simulink model "turboShaft_Harness1"  (R2024a)
settings: Solver=VariableStepAuto  StartTime=0.0  StopTime=1000  RelTol=1e-3
model workspace: external: MATLAB File C:\Users\imyrsini\OneDrive - MathWorks\Documents\Projects\AEprojects\LSTM Model Reduction\turboShaftEngine\initialization.m (data not in the file)
undefined symbols (not defined in the file): burner, height
libraries: fl_lib x1, simulink x1, nesl_utility x1
settings Model: Creator=imyrsini  LastModifiedBy=imyrsini
settings RTWCC: GPUComputeCapability=3.5
settings SimscapeCC: SimscapeLogType=all  SimscapeLogSimulationStatistics=on  SimscapeLogToSDI=on

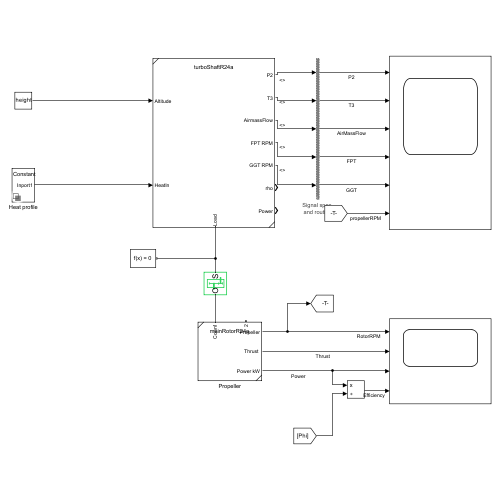
[thumbnail: Simulink's stored preview of the top-level diagram]
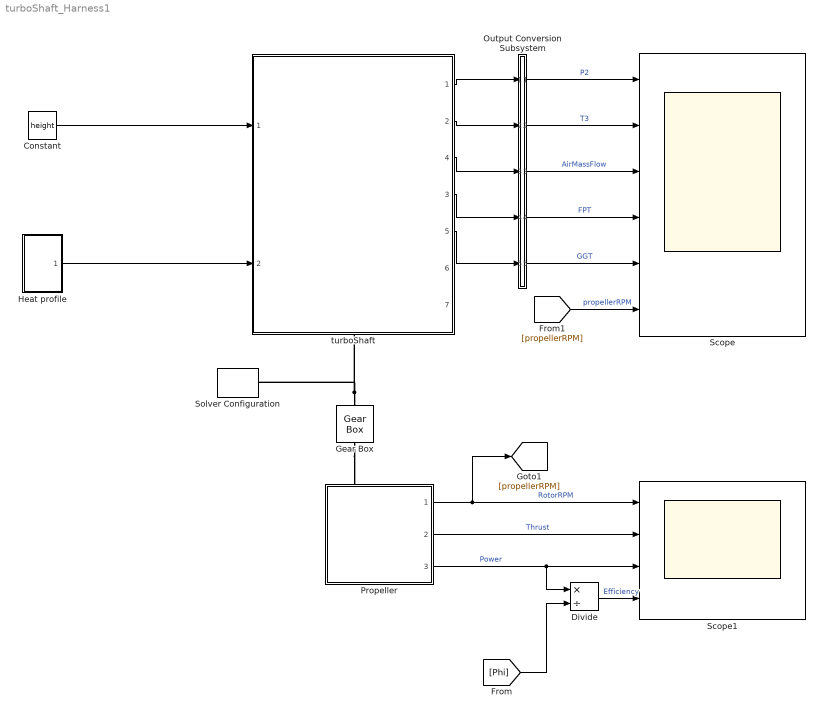
== system turboShaft_Harness1 ==
  Constant : Constant  Value=height
  Divide : Product  Inputs=*/
  Gear Box : fl_lib/Mechanical/Mechanisms/Gear Box  ratio=shaftFTP.GearRatio  t_in_specify=off  t_in_priority=None  t_in=0 N*m  t_in_nominal_specify=off  t_in_nominal_value=1  t_in_nominal_unit=N*m  t_out_specify=off  t_out_priority=None  t_out=0 N*m  t_out_nominal_specify=off  t_out_nominal_value=1  t_out_nominal_unit=N*m
  Heat profile : Subsystem  Variant=on  VariantControlMode=label  VariantControl=Choice  LabelModeActiveChoice=Choice
  Output Conversion Subsystem : Subsystem  Tag=__SLT_OCS__  Description=|
      | Signal spec.
      | and routing
      settings: AttributesFormatString=%<Description>
  Propeller : Subsystem  ReferencedSubsystem=mainRotorR24a
      settings: PortSchema="{\"entries\":[{\"content\":{\"sides\":[{\"content\":{},\"type\":\"ConnectorPlacement.EquallySpacedRectSide\",\"uuid\":\"252db255-f093-4807-9ecd-c68cc83ab3ed\"},{\"content\":{\"connectorIds\":[\"Out1\",\"Out2\",\"Out3\"],\"side\":\"RIGHT\"},\"type\":\"ConnectorPlacement.EquallySpacedRectSide\",\"uuid\":\"da666ad2-6787-4735-89e8-4b014bcd5380\"},{\"content\":{\"connectorIds\":[\"LConn1\",\"LConn2\"],\"side\":\"TOP\"},\"type\":\"ConnectorPlacement.EquallySpacedRectSide\",\"uuid\":\"73693994-4640-4975-b3ef-a4c51496569c\"}]},\"type\":\"ConnectorPlacement.EquallySpacedConnector\",\"uuid\":\"074df9fe-faaf-4ddc-9794-64f4ac4e057a\"}],\"packageUris\":[\"http://schema.mathworks.com/mf0/Connector/R2020b\"],\"version\":\"1.0\"}"
  Scope : Scope  NumInputPorts=6
  Scope1 : Scope  NumInputPorts=4
  Solver Configuration : nesl_utility/Solver Configuration  PhysicalDomain=network_engine_domain  SubClassName=solver  LeftPortType=input  RightPortType=generic  Tones=[]  Harmonics=[]  SimulateNoise=off  Profile=off  UseLocalSampling=off  EnableSwitchedLinearOptims=on  FrequencyDomain=off  UseCCode=off  RelTol=0.001  AbsTol=0.001  MinStep=1e-09  ToWorkspace=off  RevertToSquareIcSolve=off  NumHomotopyIterations=100  PhasorMode=off  PhasorModeNumHarmonics=1  ConsistencySolver=NEWTON_XTOL_AFTER_FTOL  IndexReductionMethod=DerivativeReplacement  DoDC=on  ResidualTolerance=1e-09  ConsistencyTolSource=GLOBAL  ConsistencyAbsTol=0.001  ConsistencyRelTol=0.001  ConsistencyTolFactor=0.001  UseLocalSolver=off  LocalSolverChoice=NE_BACKWARD_EULER_ADVANCER  ResolveIndetEquations=on  FunctionEvalNumThread=1  LocalSolverSampleTime=0.001  DoFixedCost=off  MaxNonlinIter=3  MaxModeIter=2  ComputeImpulses=off  ImpulseIterations=2  LinearAlgebra=auto  LinearAlgebraNumThread=0  EquationFormulation=NE_TIME_EF  DelaysMemoryBudget=1024  AutomaticFiltering=on  FilteringTimeConstant=0.001  PartitionStorageMethod=AS_NEEDED  PartitionMemoryBudget=1024  PartitionMethod=ROBUST  MultibodyUseLocalSolver=off  MultibodyLocalSolverChoice=ODE1  MultibodyLocalSolverSampleTime=0.001
  turboShaft : Subsystem  ReferencedSubsystem=turboShaftR24a
      settings: PortSchema="{\"entries\":[{\"content\":{\"sides\":[{\"content\":{\"connectorIds\":[\"In1\",\"In2\"]},\"type\":\"ConnectorPlacement.EquallySpacedRectSide\",\"uuid\":\"7ef2fcb2-1b0d-44c2-984d-f1d7df0d7e80\"},{\"content\":{\"connectorIds\":[\"Out1\",\"Out2\",\"Out4\",\"Out3\",\"Out5\",\"Out6\",\"Out7\"],\"side\":\"RIGHT\"},\"type\":\"ConnectorPlacement.EquallySpacedRectSide\",\"uuid\":\"b2d8a67b-1c6d-4b5e-865c-86345858511b\"},{\"content\":{\"side\":\"TOP\"},\"type\":\"ConnectorPlacement.EquallySpacedRectSide\",\"uuid\":\"4c7a9b07-6c1b-4859-8cda-a5c2cd89c129\"},{\"content\":{\"connectorIds\":[\"RConn1\"],\"side\":\"BOTTOM\"},\"type\":\"ConnectorPlacement.EquallySpacedRectSide\",\"uuid\":\"794a4e7c-d3e7-4ff8-9cf4-b7022afdc3bd\"}]},\"type\":\"ConnectorPlacement.EquallySpacedConnector\",\"uuid\":\"5f81fd46-9bac-4f96-9ad1-c3a7cd36c01a\"}],\"packageUris\":[\"http://schema.mathworks.com/mf0/Connector/R2020b\"],\"version\":\"1.0\"}"
  wires:
  Output Conversion Subsystem/1(Outport_1) -> Scope/1  "P2"
  Output Conversion Subsystem/2(Outport_2) -> Scope/2  "T3"
  Output Conversion Subsystem/3(Outport_3) -> Scope/3  "AirMassFlow"
  Output Conversion Subsystem/4(Outport_4) -> Scope/4  "FPT"
  Output Conversion Subsystem/5(Outport_5) -> Scope/5  "GGT"
  turboShaft/1 -> Output Conversion Subsystem/1(Inport_1)
  turboShaft/2 -> Output Conversion Subsystem/2(Inport_2)
  turboShaft/4 -> Output Conversion Subsystem/3(Inport_3)
  Propeller/1 -> [propellerRPM], Scope1/1  "RotorRPM"
  Propeller/2 -> Scope1/2  "Thrust"
  Propeller/3 -> Divide/1, Scope1/3  "Power"
  [Phi] -> Divide/2
  Divide/1 -> Scope1/4  "Efficiency"
  turboShaft/3 -> Output Conversion Subsystem/4(Inport_4)
  turboShaft/5 -> Output Conversion Subsystem/5(Inport_5)
  [propellerRPM] -> Scope/6  "propellerRPM"
  Constant/1 -> turboShaft/1
  Heat profile/1(Inport1) -> turboShaft/2
  connections:
  Gear Box/LConn1 -- Solver Configuration/RConn1 -- turboShaft/RConn1
  Gear Box/RConn1 -- Propeller/LConn1

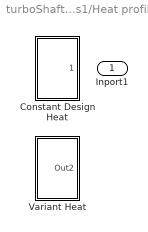
== system turboShaft_Harness1/Heat profile ==
  Constant Design Heat : Subsystem  VariantControl=Choice
  Variant Heat : Subsystem  VariantControl=Choice_1
  Inport1 : Outport

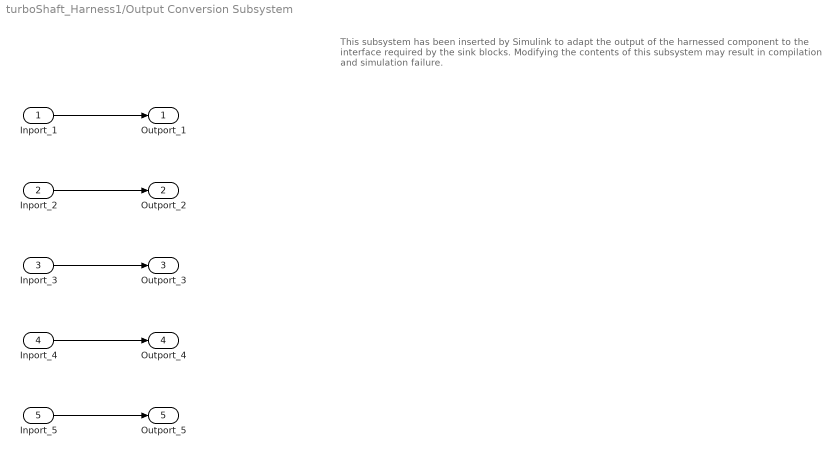
== system turboShaft_Harness1/Output Conversion Subsystem ==
  note: This subsystem has been inserted by Simulink to adapt the output of the harnessed component to the interface required by the sink blocks.
      |  Modifying the contents of this subsystem may result in compilation and simulation failure.
  Inport_1 : Inport
  Inport_2 : Inport  Port=2
  Inport_3 : Inport  Port=3
  Inport_4 : Inport  Port=4
  Inport_5 : Inport  Port=5
  Outport_1 : Outport
  Outport_2 : Outport  Port=2
  Outport_3 : Outport  Port=3
  Outport_4 : Outport  Port=4
  Outport_5 : Outport  Port=5
  wires:
  Inport_1/1 -> Outport_1/1
  Inport_2/1 -> Outport_2/1
  Inport_3/1 -> Outport_3/1
  Inport_4/1 -> Outport_4/1
  Inport_5/1 -> Outport_5/1

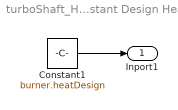
== system turboShaft_Harness1/Heat profile/Constant Design Heat ==
  Constant1 : Constant  Value=burner.heatDesign
  Inport1 : Outport
  wires:
  Constant1/1 -> Inport1/1

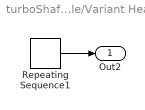
== system turboShaft_Harness1/Heat profile/Variant Heat ==
  Repeating Sequence1 : simulink/Sources/Repeating Sequence  rep_seq_t=[0 100 150 250 300 400 450 550 600 700 750 850 900 1100]  rep_seq_y=[1e3 1e3 2e3 2e3 3e3 3e3 4e3 4e3 5e3 5e3 6e3 6e3 7e3 7e3]
  Out2 : Outport
  wires:
  Repeating Sequence1/1 -> Out2/1
